simulink model "compartmentModel"  (R2020b)
settings: Solver=VariableStepAuto  StartTime=0.0  StopTime=5.00  RelTol=1e-3
libraries: simulink x1
settings Model: Creator=zsj24  LastModifiedBy=zsj24

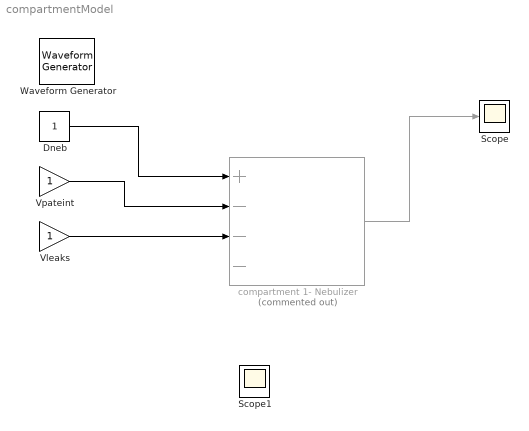
== system compartmentModel ==
  Dneb : Constant
  Scope : Scope
  Scope1 : Scope
  Vleaks : Gain
  Vpateint : Gain
  Waveform Generator : simulink/Sources/Waveform Generator  OutMin=[]  OutMax=[]  OutDataTypeStr=double  SelectedSignal=1  BlockNames=MultiportSwitch_e3df3653d217406  SampleTime=0.1
  compartment 1- Nebulizer : Sum  Commented=on  Inputs=+---
  wires:
  Vleaks/1 -> compartment 1- Nebulizer/3
  Dneb/1 -> compartment 1- Nebulizer/1
  compartment 1- Nebulizer/1 -> Scope/1
  Vpateint/1 -> compartment 1- Nebulizer/2
